simulink model "friction_logData"  (R2017a)
settings: Solver=VariableStepAuto  StartTime=0.0  StopTime=20  RelTol=1e-3
values from neighbouring files (symbols this model uses):
  Fc = 0.58    [Script_Friction.m]
  Fs = 1    [Script_Friction.m]
  i = 2    [Script_Friction.m]
  kv = 1    [Script_Friction.m]
  sigma0 = 2000    [Script_Friction.m]
  sigma1 = 1000    [Script_Friction.m]
  sigma2 = 1.295    [Script_Friction.m]    (also in sim_dynamic_param_full_identif.m; sim_dynamic_param_identif.m; sim_dynamic_param_identify_LS.m)
  vs = 0.001    [Script_Friction.m]
libraries: simulink x6
settings Model: Creator=igricart  LastModifiedBy=igricart

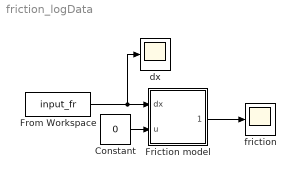
== system friction_logData ==
  Constant : Constant  Value=0
  Friction model : Subsystem
  From Workspace : FromWorkspace  VariableName=input_fr  SampleTime=0
  dx : Scope
  friction : Scope
  wires:
  From Workspace/1 -> dx/1, Friction model/1(dx)
  Friction model/1(Friction) -> friction/1
  Constant/1 -> Friction model/2(u)

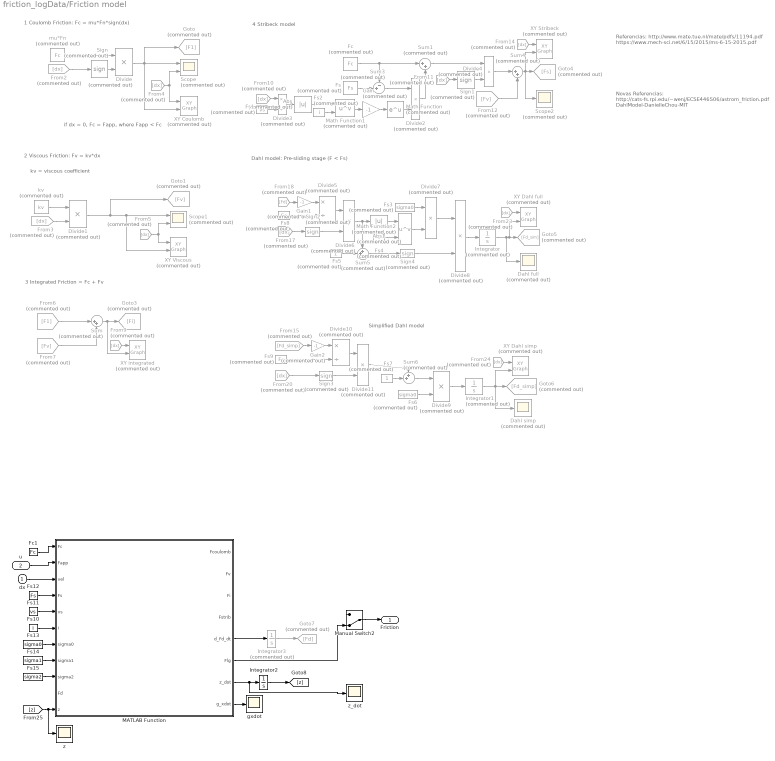
== system friction_logData/Friction model ==
  note: Novas Referencias:
      | http://cats-fs.rpi.edu/~wenj/ECSE446S06/astrom_friction.pdf
      | DahlModel-DanielleChou-MIT
  note: Simplified Dahl model
  note: Dahl model: Pre-sliding stage (F < Fs)
  note: 4 Stribeck model
  note: 3 Integrated Friction = Fc + Fv
  note: if dx = 0, Fc = Fapp, where Fapp < Fc
  note: kv = viscous coefficient
  note: Referencias:
      | http://www.mate.tue.nl/mate/pdfs/11194.pdf
      | https://www.mech-sci.net/6/15/2015/ms-6-15-2015.pdf
  note: 1 Coulomb Friction: Fc = mu*Fn*sign(dx)
  note: 2 Viscous Friction: Fv = kv*dx
  dx : Inport
  u : Inport  Port=2
  Abs : Abs  Commented=on
  Abs1 : Abs  Commented=on
  Dahl full : Scope  Commented=on
  Dahl simp : Scope  Commented=on
  Divide{,1..2,4,6..9,11} (9 alike) : Product  Commented=on  Inputs=**
  Divide10 : Product  Commented=on  Inputs=*/
  Divide3 : Product  Commented=on  Inputs=*/
  Divide5 : Product  Commented=on  Inputs=*/
  Fc : Constant  Commented=on  Value=Fc
  Fc1 : Constant  Value=Fc
  From{2..5,9..11,14,17,20,23..24} (12 alike) : From  Commented=on  GotoTag=dx
  From12 : From  Commented=on  GotoTag=Fv
  From15 : From  Commented=on  GotoTag=Fd_simp
  From18 : From  Commented=on  GotoTag=Fd
  From6 : From  Commented=on  GotoTag=F1
  From7 : From  Commented=on  GotoTag=Fv
  Fs : Constant  Commented=on  Value=Fs
  Fs1 : Constant  Commented=on  Value=vs
  Fs10 : Constant  Value=i
  Fs11 : Constant  Value=vs
  Fs12 : Constant  Value=Fs
  Fs13 : Constant  Value=sigma0
  Fs14 : Constant  Value=sigma1
  Fs15 : Constant  Value=sigma2
  Fs2 : Constant  Commented=on  Value=i
  Fs3 : Constant  Commented=on  Value=sigma0
  Fs4 : Constant  Commented=on  Value=i
  Fs5 : Constant  Commented=on
  Fs6 : Constant  Commented=on  Value=sigma0
  Fs7 : Constant  Commented=on
  Fs8 : Constant  Commented=on  Value=Fc
  Fs9 : Constant  Commented=on  Value=Fc
  Gain : Gain  Commented=on  Gain=-1
  Gain1 : Gain  Commented=on  Gain=-1
  Gain2 : Gain  Commented=on  Gain=-1
  Goto : Goto  Commented=on  GotoTag=F1
  Goto1 : Goto  Commented=on  GotoTag=Fv
  Goto3 : Goto  Commented=on  GotoTag=Fi
  Goto4 : Goto  Commented=on  GotoTag=Fs
  Goto5 : Goto  Commented=on  GotoTag=Fd_sim
  Goto6 : Goto  Commented=on  GotoTag=Fd_simp
  Goto7 : Goto  Commented=on  GotoTag=Fd
  Integrator : Integrator  Commented=on  InitialCondition=Fc
  Integrator1 : Integrator  Commented=on  InitialCondition=Fc
  Integrator2 : Integrator
  Integrator3 : Integrator  Commented=on
  MATLAB Function : MATLAB Function  TreatAsAtomicUnit=on
  Manual Switch2 : ManualSwitch  CurrentSetting=0
  Math Function : Math  Commented=on  SaturateOnIntegerOverflow=on
  Math Function1 : Math  Commented=on  Operator=pow  SaturateOnIntegerOverflow=on
  Math Function2 : Math  Commented=on  Operator=pow  SaturateOnIntegerOverflow=on
  Scope : Scope  Commented=on  NumInputPorts=2
  Scope1 : Scope  Commented=on  NumInputPorts=2
  Scope2 : Scope  Commented=on
  Sign{,1..4} (5 alike) : Signum  Commented=on
  Sum : Sum  Commented=on  Inputs=|++
  Sum1 : Sum  Commented=on  Inputs=|++
  Sum3 : Sum  Commented=on  Inputs=-+|
  Sum4 : Sum  Commented=on  Inputs=|++
  Sum5 : Sum  Commented=on  Inputs=++|
  Sum6 : Sum  Commented=on  Inputs=++|
  XY Coulomb : simulink/Sinks/XY Graph  Commented=on  xmin=-0.15  xmax=0.15  ymin=-15  ymax=15  st=-1
  XY Dahl full : simulink/Sinks/XY Graph  Commented=on  xmin=-0.2  xmax=0.2  ymin=0  ymax=5  st=-1
  XY Dahl simp : simulink/Sinks/XY Graph  Commented=on  xmin=-0.15  xmax=0.15  ymin=-15  ymax=15  st=-1
  XY Stribeck : simulink/Sinks/XY Graph  Commented=on  xmin=-0.15  xmax=0.15  ymin=-15  ymax=15  st=-1
  XY Viscous : simulink/Sinks/XY Graph  Commented=on  xmin=-0.15  xmax=0.15  ymin=-15  ymax=15  st=-1
  XY integrated : simulink/Sinks/XY Graph  Commented=on  xmin=-0.15  xmax=0.15  ymin=-15  ymax=15  st=-1
  gxdot : Scope
  kv : Constant  Commented=on  Value=kv
  mu*Fn : Constant  Commented=on  Value=Fc
  z : Scope
  z_dot : Scope
  Friction : Outport
  wires:
  Sign/1 -> Divide/2
  mu*Fn/1 -> Divide/1
  kv/1 -> Divide1/1
  From2/1 -> Sign/1
  Divide1/1 -> XY Viscous/2, Scope1/1, Goto1/1
  From3/1 -> Divide1/2
  Divide/1 -> XY Coulomb/2, Goto/1, Scope/1
  From4/1 -> Scope/2, XY Coulomb/1
  From5/1 -> XY Viscous/1, Scope1/2
  From6/1 -> Sum/1
  From7/1 -> Sum/2
  Sum/1 -> XY integrated/2, Goto3/1
  From9/1 -> XY integrated/1
  Fc/1 -> Sum3/1, Sum1/1
  Fs/1 -> Sum3/2
  Sum3/1 -> Divide2/1
  Math Function/1 -> Divide2/2
  From10/1 -> Divide3/1
  Fs1/1 -> Divide3/2
  Divide3/1 -> Abs/1
  Math Function1/1 -> Gain/1
  Fs2/1 -> Math Function1/2
  Gain/1 -> Math Function/1
  Abs/1 -> Math Function1/1
  Divide2/1 -> Sum1/2
  Sign1/1 -> Divide4/2
  From11/1 -> Sign1/1
  Sum1/1 -> Divide4/1
  Divide4/1 -> Sum4/1
  From12/1 -> Sum4/2
  Sum4/1 -> Scope2/1, XY Stribeck/2, Goto4/1
  From14/1 -> XY Stribeck/1
  From17/1 -> Sign2/1
  Fs8/1 -> Divide5/2
  From18/1 -> Gain1/1
  Gain1/1 -> Divide5/1
  Divide5/1 -> Divide6/1
  Sign2/1 -> Divide6/2
  Divide6/1 -> Sum5/1, Abs1/1
  Fs4/1 -> Math Function2/2
  Abs1/1 -> Math Function2/1
  Math Function2/1 -> Divide7/2
  Fs3/1 -> Divide7/1
  Divide7/1 -> Divide8/1
  Sum5/1 -> Sign4/1
  Divide8/1 -> Integrator/1
  Fs6/1 -> Divide9/2
  Fs5/1 -> Sum5/2
  Divide9/1 -> Integrator1/1
  Fs7/1 -> Sum6/2
  Sum6/1 -> Divide9/1
  Divide11/1 -> Sum6/1
  Sign3/1 -> Divide11/2
  Divide10/1 -> Divide11/1
  Gain2/1 -> Divide10/1
  From15/1 -> Gain2/1
  Fs9/1 -> Divide10/2
  From20/1 -> Sign3/1
  Integrator/1 -> Dahl full/1, XY Dahl full/2, Goto5/1
  From23/1 -> XY Dahl full/1
  From24/1 -> XY Dahl simp/1
  Integrator1/1 -> Dahl simp/1, XY Dahl simp/2, Goto6/1
  Sign4/1 -> Divide8/2
  dx/1 -> MATLAB Function/3(vel)
  Fs10/1 -> MATLAB Function/6(i)
  Fs11/1 -> MATLAB Function/5(vs)
  Fs12/1 -> MATLAB Function/4(Fs)
  Fc1/1 -> MATLAB Function/1(Fc)
  Fs13/1 -> MATLAB Function/7(sigma0)
  Integrator3/1 -> Goto7/1
  ? -> MATLAB Function/10(Fd)
  Integrator2/1 -> [z]
  MATLAB Function/7(z_dot) -> z_dot/1, Integrator2/1
  Fs14/1 -> MATLAB Function/8(sigma1)
  Fs15/1 -> MATLAB Function/9(sigma2)
  [z] -> z/1, MATLAB Function/11(z)
  MATLAB Function/6(Flg) -> Manual Switch2/2
  MATLAB Function/5(d_Fd_dt) -> Integrator3/1
  Manual Switch2/1 -> Friction/1
  u/1 -> MATLAB Function/2(Fapp)
  MATLAB Function/8(g_xdot) -> gxdot/1

== matlab function friction_logData/Friction model/MATLAB Function ==
  data: Fcoulomb output; Fc input; Fapp input; vel input; Fs input; vs input; i input; sigma0 input; sigma1 input; sigma2 input; Fv output; Fi output; Fstrib output; Fd input; d_Fd_dt output; Flg output; z_dot output; z input; g_xdot output
%% Function with friction models

function [Fcoulomb ,Fv ,Fi ,Fstrib ,d_Fd_dt ,Flg ,z_dot,g_xdot] = friction(Fc ,Fapp ,vel ,Fs ,vs ,i ,sigma0 ,sigma1 ,sigma2 ,Fd ,z)

%% Coulomb Friction and Viscous Friction
if vel ~= 0
    Fcoulomb = Fc*sign(vel);
    Fv = sigma2*vel + Fcoulomb;
elseif abs(Fapp) < Fs
    Fcoulomb = Fapp;
    Fv = Fcoulomb;
else %v == 0 && abs(Fapp) >= Fs
    Fcoulomb = Fc*sign(Fapp);
    Fv = Fcoulomb;
end
   
%% Integrated Coulomb Friction and Viscous Friction with friction force
% transition
if (vel >= 0)
    Fi = min(Fc,Fv);
else
    Fi = max(-Fc,Fv);
end

%% Stribeck model
F = (Fc + (Fs - Fc) * exp(-(abs(vel/vs))^i)) * sign(vel) + Fv;

if vel ~= 0
    Fstrib = F;
elseif abs(Fapp) < Fs
    Fstrib = Fapp;
else %v == 0 && abs(Fapp) >= Fs
    Fstrib = Fs*sign(Fapp);
end

%% Dahl Model - Pre-sliding (Fd < Fs)
% d_Fd_dx = sigma0 * (abs(1 - Fd/Fc * sign(vel)))^i * sign(1 - Fd / Fc * sign(vel));
d_Fd_dx = sigma0 * (abs(1 - Fd/Fc * sign(vel)))^i;

%Simplified model where i = 1
%d_Fd_dx_mod = sigma0 * (1 - Fd/Fc * sign(vel));

% OBs.: d_Fd_dt  = d_Fd_dx * dx_dt
d_Fd_dt = d_Fd_dx * vel;
%% LeGru model
% Alpeter dc thesis
% Normally i  =  2
% g_xdot = Fc + (Fs - Fc) * exp(-(abs(vel/vs))^i);
% z_dot = vel - sigma0 * vel * z / g_xdot;
% Flg = sigma0 * z + sigma1 * z_dot + sigma2 * vel;

%Astrom paper
% Variable damping coefficient decreasing with increasing velocity
vd = 1e-1; 
sigma1_v = sigma1*exp(-(vel/vd)^2);

% Olsson paper
g_xdot = Fc + (Fs - Fc) * exp(-i*abs(vel));
z_dot = vel - sigma0 * abs(vel) * z / g_xdot;
Flg = sigma0 * z + sigma1 * z_dot + sigma2 * vel;
